simulink model "Exp_3_9"  (R2024b)
settings: Solver=VariableStepAuto  StartTime=0.0  StopTime=10.0  RelTol=1e-3
settings Model: Creator=Rj Avro Biswas  LastModifiedBy=Rj Avro Biswas

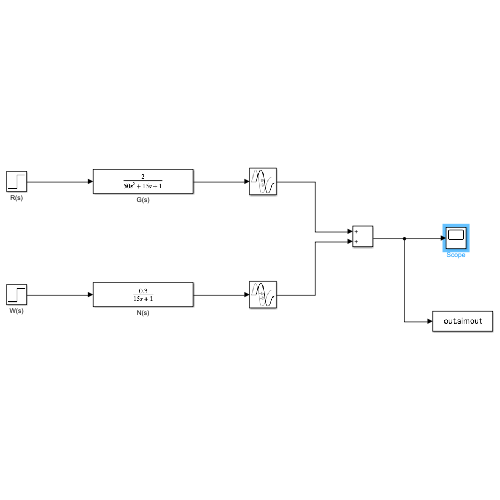
[thumbnail: Simulink's stored preview of the top-level diagram]
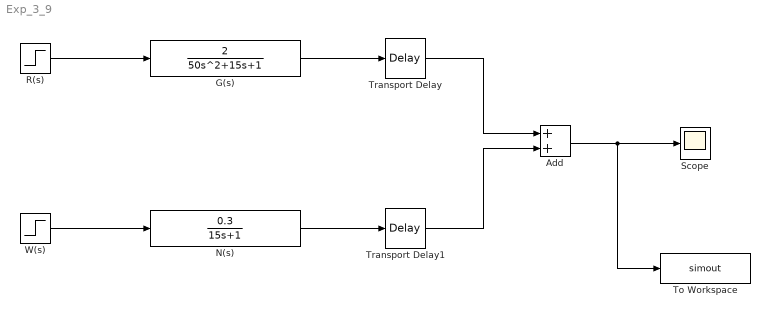
== system Exp_3_9 ==
  Add : Sum
  G(s) : TransferFcn  Numerator=[2]  Denominator=[50 15 1]
  N(s) : TransferFcn  Numerator=[0.3]  Denominator=[15 1]
  R(s) : Step  SampleTime=0
  Scope : Scope
  To Workspace : ToWorkspace  VariableName=simout  SaveFormat=Timeseries  SampleTime=-1
  Transport Delay : TransportDelay  DelayTime=exp(-5)
  Transport Delay1 : TransportDelay  DelayTime=exp(-5)
  W(s) : Step  SampleTime=0
  wires:
  W(s)/1 -> N(s)/1
  R(s)/1 -> G(s)/1
  G(s)/1 -> Transport Delay/1
  Transport Delay/1 -> Add/1
  Transport Delay1/1 -> Add/2
  N(s)/1 -> Transport Delay1/1
  Add/1 -> To Workspace/1, Scope/1
